simulink model "integratoin_2"  (R2023b)
settings: Solver=FixedStepAuto  StartTime=0.0  StopTime=inf  FixedStep=Ts  RelTol=1e-3
InitFcn:
  | params
  | pin_params
undefined symbols (not defined in the file): b, den_Gd, encoder_scale, f, J, Kb, KD, Kf, KI, Km, KP, l, L, num_Gd, r, R, Vlim, Wref
libraries: arduinolib x29, arduinosensorlib x12, simulink x8
(part 2 of 2)

== stateflow chart integratoin_2/Chart ==
  state AccOff
    en: state=state+1;
    v1=sw1;
    v2=sw2;
    n=state/100
    du:
  state AccStandby
    en: state=state+1;
    v1=sw1;
    v2=sw2;
    n=state/100
    du:
  state AccOn1
    en: state=state-1;
    v1=sw1;
    v2=sw2;
    n=state/100
    du:
  state AccOn
    en: state=state-1;
    v1=sw1;
    v2=sw2;
    n=state/100
    du:
  (default) -> AccOff : {state=-1}
  AccOff -> AccStandby [order 1] : [v1~=sw1]
  AccStandby -> AccOff [order 1] : [v1~=sw1]
  AccOff -> AccOn [order 2] : [v2~=sw2]
  AccOn -> AccOff [order 2] : [v1~=sw1]
  AccOn1 -> AccStandby [order 1] : [v1~=sw1]
  AccStandby -> AccOn1 [order 2] : [v2~=sw2]
  AccOn1 -> AccOn [order 2] : [v2~=sw2]
  AccOn -> AccOn1 [order 1] : [v2~=sw2]
  data: sw1 input; v1 local; v2 local; sw2 input; n output; state local

== stateflow chart integratoin_2/Subsystem13/Chart ==
  state drive_on_adas_on
    en, du:
    out1 = default;
    out2 = default;
  state drive_off
    en, du:
    out1 = 0;
    out2 = 0;
    steering = 0.02;
    default = 360;
  state drive_on_adas_off
    en, du:
    out1 = default*(1+(handle-128)/6.4/100);
    out2 = default*(1+(128-handle)/6.4/100);
    exit:
    buzzer = 0;
  state drive_on_adas_on_FUS
    en,du:
    out1 = 0;
    out2 = 0;
    buzzer = 1;
    exit:
    buzzer = 0;
  state drive_on_adas_on_LUS
    en,du:
    out1 = default*(1+(10-LUS)*steering);
    out2 = default*(1-(10-LUS)*steering);
  state drive_on_adas_on_RUS
    en,du:
    out1 = default*(1-(10-RUS)*steering);
    out2 = default*(1+(10-RUS)*steering);
  state drive_on_adas_on_LRUS
    en,du:
    out1 = default*(1-(LUS-RUS)*steering);
    out2 = default*(1+(LUS-RUS)*steering);
  drive_on_adas_on_FUS -> drive_on_adas_off [order 5] : [adas_mode ==0]
  (default) -> drive_off
  drive_on_adas_on -> drive_on_adas_on_FUS [order 2] : [FUS<=10]
  drive_on_adas_on_FUS -> drive_on_adas_on_LUS [order 4] : [LUS<=10&&FUS>10]
  drive_off -> drive_on_adas_off : [drive_mode==1]
  drive_on_adas_off -> drive_on_adas_on [order 2] : [adas_mode == 1]
  drive_on_adas_on_FUS -> drive_on_adas_on [order 1] : [LUS>10&&RUS>10&&FUS>10]
  drive_on_adas_off -> drive_off [order 1] : [drive_mode ==0]
  drive_on_adas_on_FUS -> drive_on_adas_on_LRUS [order 2] : [LUS<=10&&RUS<=10&&FUS>10]
  drive_on_adas_on -> drive_on_adas_off [order 1] : [adas_mode  == 0]
  drive_on_adas_on_RUS -> drive_on_adas_off [order 4] : [adas_mode ==0]
  drive_on_adas_on -> drive_on_adas_on_LUS [order 4] : [LUS<=10]
  drive_on_adas_on_LUS -> drive_on_adas_on [order 1] : [LUS>10]
  drive_on_adas_on -> drive_on_adas_on_RUS [order 3] : [RUS<=10]
  drive_on_adas_on_RUS -> drive_on_adas_on [order 1] : [RUS>10]
  drive_on_adas_on_LUS -> drive_on_adas_off [order 4] : [adas_mode ==0]
  drive_on_adas_on_LRUS -> drive_on_adas_off [order 4] : [adas_mode==0]
  drive_on_adas_on_LUS -> drive_on_adas_on_FUS [order 3] : [FUS<=10]
  drive_on_adas_on_LRUS -> drive_on_adas_on_FUS [order 1] : [FUS<=10]
  drive_on_adas_on_RUS -> drive_on_adas_on_FUS [order 2] : [FUS<=10]
  drive_on_adas_on_FUS -> drive_on_adas_on_RUS [order 3] : [RUS<=10&&FUS>10]
  drive_on_adas_on_RUS -> drive_on_adas_on_LRUS [order 3] : [LUS<=10]
  drive_on_adas_on_LRUS -> drive_on_adas_on_RUS [order 3] : [LUS>10]
  drive_on_adas_on_LUS -> drive_on_adas_on_LRUS [order 2] : [RUS<=10]
  drive_on_adas_on_LRUS -> drive_on_adas_on_LUS [order 2] : [RUS>10]
  data: drive_mode input; adas_mode input; FUS input; LUS input; RUS input; out1 output; out2 output; handle input double; buzzer output; steering local double; speed1 local double; speed2 local double; default local double

== stateflow chart integratoin_2/Subsystem13/Chart1 ==
  state adas_off
    en,du:
    rout1=out1;
    rout2=out2;
  state adas_on
    en,du:
    rout1=out1;
    rout2=out2;
  state adas_on_BUS
    en,du:
    rout1=out1*1.2;
    rout2=out2*1.2;
  adas_on_BUS -> adas_off [order 2] : [adas_mode==0]
  (default) -> adas_off
  adas_on -> adas_on_BUS [order 2] : [BUS<=10]
  adas_off -> adas_on : [adas_mode==1]
  adas_on -> adas_off [order 1] : [adas_mode==0]
  adas_on_BUS -> adas_on [order 1] : [BUS>10]
  data: adas_mode input; out1 input; out2 input; BUS input; rout1 output; rout2 output

== stateflow chart integratoin_2/light_Ctrl/Subsystem/Chart1 ==
  state light_auto
    en, du:
    light_mode = 1;
    state_1 = sw3;
  state light_off
    en, du:
    light_mode =0;
    state_1 = sw3;
  state light_on
    en,du:
    light_mode =2;
    state_1 = sw3;
  light_auto -> (junction 15) : [(state_1 ~= sw3) && (Drive_mode == 1)]
  (junction 12) -> light_auto
  (junction 15) -> light_on
  light_off -> (junction 12) : [(state_1 ~= sw3) && (Drive_mode == 1)]
  (default) -> light_off
  light_on -> light_off : [(state_1 ~= sw3) && (Drive_mode == 1)]
  data: sw3 input; Drive_mode input; state_1 local; light_mode output

== stateflow chart integratoin_2/State_Ctrl/ADAS_state/If Action Subsystem/Chart ==
  state adas_off
    en,du:
    ADAS_state = sw2;
    state_2 = sw2;
  state adas_on
    en,du:
    ADAS_state = sw2;
    state_2 =sw2;
  (default) -> adas_off
  adas_off -> adas_on : [state_2 ~= sw2]
  adas_on -> adas_off : [state_2 ~= sw2]
  data: sw2 input; state_2 local; ADAS_state output

== stateflow chart integratoin_2/State_Ctrl/drive_mode/Chart ==
  state Drive_off
    en, du:
    drive_mode = 0;
    state_1 = sw1;
  state Drive_on
    en,du:
    drive_mode =1;
    state_1 = sw1;
    ADAS_state = A_state;
    Light_state = light_mode;
  (default) -> Drive_off
  Drive_off -> Drive_on : [state_1 ~= sw1]
  Drive_on -> Drive_off : [(state_1~=sw1) && (ADAS_state == 0) && (Light_state == 0)]
  data: sw1 input; light_mode input; state_1 local; drive_mode output; A_state input; ADAS_state local; Light_state local
